simulink model "test_sim"  (Simulink 10.3)
settings: Solver=ode4  StartTime=0.0  StopTime=1  FixedStep=0.001  RelTol=1e-3  EnableMultiTasking=on
settings Model: Creator=ljk  LastModifiedBy=fu  ExtModeTrigMode=oneshot  ExtModeArmWhenConnect=off
settings OptimizationCC: BlockReduction=off  BooleanDataType=off
settings DebuggingCC: SaveWithParameterizedLinksMsg=none  SignalResolutionControl=TryResolveAllWithWarning  MultiTaskDSMMsg=warning  MultiTaskCondExecSysMsg=none
settings HardwareCC: TargetUnknown=on

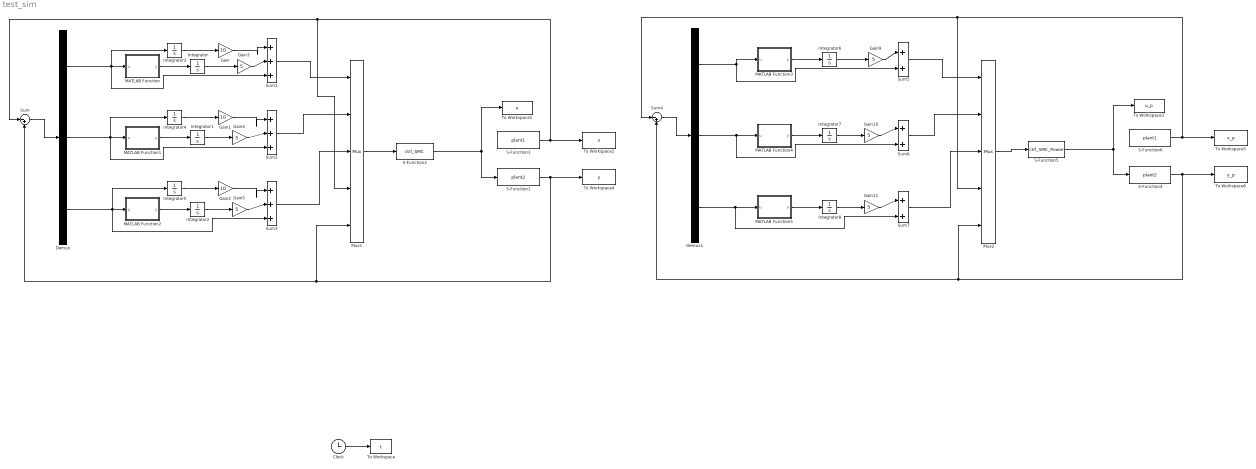
== system test_sim ==
  Clock : Clock
  Demux : Demux  Outputs=3
  Demux1 : Demux  Outputs=3
  Gain : Gain  Gain=10
  Gain1 : Gain  Gain=10
  Gain{3..5,9..11} (6 alike) : Gain  Gain=5
  Gain2 : Gain  Gain=10
  Integrator{,1..8} (9 alike) : Integrator
  MATLAB Function : MATLAB Function  TreatAsAtomicUnit=on
  MATLAB Function1 : MATLAB Function  TreatAsAtomicUnit=on
  MATLAB Function2 : MATLAB Function  TreatAsAtomicUnit=on
  MATLAB Function3 : MATLAB Function  TreatAsAtomicUnit=on
  MATLAB Function4 : MATLAB Function  TreatAsAtomicUnit=on
  MATLAB Function5 : MATLAB Function  TreatAsAtomicUnit=on
  Mux1 : Mux  Inputs=5
  Mux2 : Mux  Inputs=5
  S-Function1 : S-Function  FunctionName=plant2  SFunctionDeploymentMode=off  EnableBusSupport=off
  S-Function2 : S-Function  FunctionName=ctrl_SMC  SFunctionDeploymentMode=off  EnableBusSupport=off
  S-Function3 : S-Function  FunctionName=plant1  SFunctionDeploymentMode=off  EnableBusSupport=off
  S-Function4 : S-Function  FunctionName=plant2  SFunctionDeploymentMode=off  EnableBusSupport=off
  S-Function5 : S-Function  FunctionName=ctrl_SMC_Power  SFunctionDeploymentMode=off  EnableBusSupport=off
  S-Function6 : S-Function  FunctionName=plant1  SFunctionDeploymentMode=off  EnableBusSupport=off
  Sum : Sum  Inputs=|-+
  Sum1 : Sum  Inputs=|+++
  Sum2 : Sum  Inputs=|+++
  Sum3 : Sum  Inputs=|+++
  Sum4 : Sum  Inputs=|-+
  Sum5 : Sum  Inputs=|++
  Sum6 : Sum  Inputs=|++
  Sum7 : Sum  Inputs=|++
  To Workspace : ToWorkspace  VariableName=t  SampleTime=-1
  To Workspace1 : ToWorkspace  VariableName=u  SampleTime=-1
  To Workspace2 : ToWorkspace  VariableName=x  SampleTime=-1
  To Workspace3 : ToWorkspace  VariableName=u_p  SampleTime=-1
  To Workspace4 : ToWorkspace  VariableName=y  SampleTime=-1
  To Workspace5 : ToWorkspace  VariableName=x_p  SampleTime=-1
  To Workspace6 : ToWorkspace  VariableName=y_p  SampleTime=-1
  wires:
  Clock/1 -> To Workspace/1
  S-Function2/1 -> S-Function1/1, To Workspace1/1
  S-Function1/1 -> To Workspace4/1, Mux1/5, Sum/2
  S-Function3/1 -> Mux1/4, Sum/1, To Workspace2/1
  Sum/1 -> Demux/1
  MATLAB Function/1(y) -> Integrator/1
  MATLAB Function1/1(y) -> Integrator1/1
  MATLAB Function2/1(y) -> Integrator2/1
  Demux/1 -> Sum1/3, MATLAB Function/1(u), Integrator3/1
  Demux/3 -> Sum3/3, Integrator5/1, MATLAB Function2/1(u)
  Demux/2 -> Sum2/3, Integrator4/1, MATLAB Function1/1(u)
  Integrator/1 -> Gain3/1
  Integrator3/1 -> Gain/1
  Integrator4/1 -> Gain1/1
  Integrator1/1 -> Gain4/1
  Integrator5/1 -> Gain2/1
  Integrator2/1 -> Gain5/1
  Gain/1 -> Sum1/1
  Gain3/1 -> Sum1/2
  Gain4/1 -> Sum2/2
  Gain1/1 -> Sum2/1
  Gain2/1 -> Sum3/1
  Gain5/1 -> Sum3/2
  Sum1/1 -> Mux1/1
  Sum2/1 -> Mux1/2
  Sum3/1 -> Mux1/3
  Mux1/1 -> S-Function2/1
  Integrator6/1 -> Gain9/1
  Integrator7/1 -> Gain10/1
  Sum7/1 -> Mux2/3
  Mux2/1 -> S-Function5/1
  Demux1/3 -> Sum7/2, MATLAB Function5/1(u)
  Sum4/1 -> Demux1/1
  MATLAB Function4/1(y) -> Integrator7/1
  Demux1/2 -> Sum6/2, MATLAB Function4/1(u)
  Sum6/1 -> Mux2/2
  Integrator8/1 -> Gain11/1
  S-Function6/1 -> Mux2/4, Sum4/1, To Workspace5/1
  Sum5/1 -> Mux2/1
  MATLAB Function3/1(y) -> Integrator6/1
  S-Function5/1 -> S-Function4/1, To Workspace3/1
  S-Function4/1 -> To Workspace6/1, Mux2/5, Sum4/2
  Demux1/1 -> Sum5/2, MATLAB Function3/1(u)
  MATLAB Function5/1(y) -> Integrator8/1
  Gain9/1 -> Sum5/1
  Gain10/1 -> Sum6/1
  Gain11/1 -> Sum7/1

== matlab function MATLAB Function1 ==
  data: u input double; y output double
function y = fcn(u)

y = u/(abs(u)+0.001);

== matlab function MATLAB Function ==
  data: u input double; y output double
function y = fcn(u)

y = u/(abs(u)+0.001);

== matlab function MATLAB Function2 ==
  data: u input double; y output double
function y = fcn(u)

y = u/(abs(u)+0.001);

== matlab function MATLAB Function3 ==
  data: u input double; y output double
function y = fcn(u)

y = abs(u)^(0.6)*u/(abs(u)+0.001);

== matlab function MATLAB Function4 ==
  data: u input double; y output double
function y = fcn(u)

y = abs(u)^(0.6)*u/(abs(u)+0.001);

== matlab function MATLAB Function5 ==
  data: u input double; y output double
function y = fcn(u)

y = abs(u)^(0.6)*u/(abs(u)+0.001);
